simulink model "LRSim1D_V3"  (R2016b)
settings: Solver=ode45  StartTime=0  StopTime=tend  FixedStep=0.005  RelTol=1e-4
values from neighbouring files (symbols this model uses):
  g = 9.81    [EnginePerformance.m]    (also in LaunchControl.m; runsim.m)
undefined symbols (not defined in the file or in its folder): Eng, Prop, Roc
settings Model: Creator=adamb  LastModifiedBy=adamb
settings SolverCC: ZeroCrossAlgorithm=Adaptive

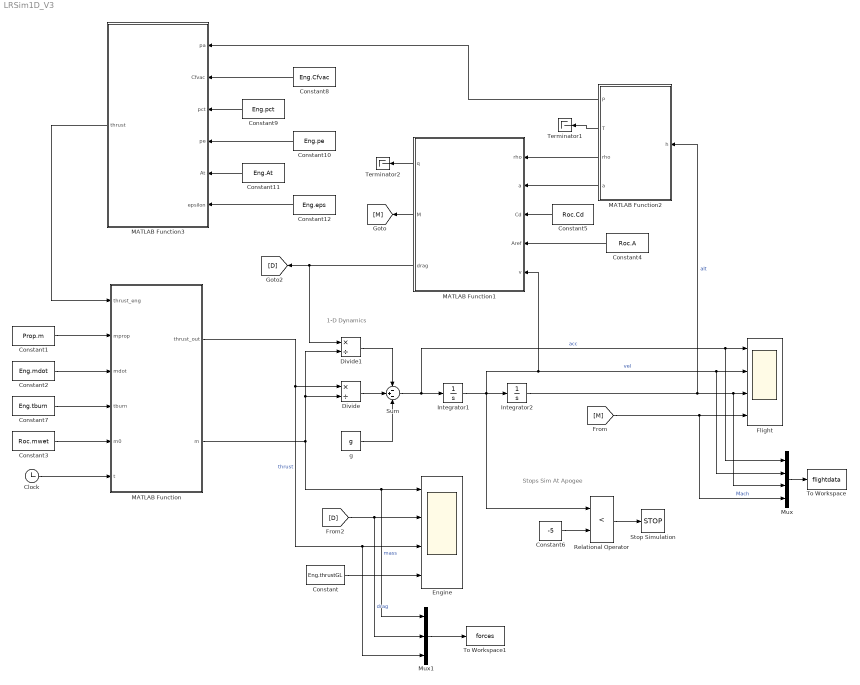
== system LRSim1D_V3 ==
  note: Stops Sim At Apogee
  note: 1-D Dynamics
  Clock : Clock
  Constant : Constant  Value=Eng.thrustGL
  Constant1 : Constant  Value=Prop.m
  Constant10 : Constant  Value=Eng.pe
  Constant11 : Constant  Value=Eng.At
  Constant12 : Constant  Value=Eng.eps
  Constant2 : Constant  Value=Eng.mdot
  Constant3 : Constant  Value=Roc.mwet
  Constant4 : Constant  Value=Roc.A
  Constant5 : Constant  Value=Roc.Cd  VectorParams1D=off
  Constant6 : Constant  Value=-5
  Constant7 : Constant  Value=Eng.tburn
  Constant8 : Constant  Value=Eng.Cfvac
  Constant9 : Constant  Value=Eng.pct
  Divide : Product  Inputs=*/
  Divide1 : Product  Inputs=*/
  Engine : Scope  NumInputPorts=4
  Flight : Scope  NumInputPorts=4
  Integrator1 : Integrator
  Integrator2 : Integrator
  MATLAB Function : MATLAB Function  TreatAsAtomicUnit=on
  MATLAB Function1 : MATLAB Function  TreatAsAtomicUnit=on
  MATLAB Function2 : MATLAB Function  TreatAsAtomicUnit=on
  MATLAB Function3 : MATLAB Function  TreatAsAtomicUnit=on
  Mux : Mux
  Mux1 : Mux  Inputs=3
  Relational Operator : RelationalOperator  Operator=<  OutDataTypeStr=boolean  RndMeth=Simplest
  Stop Simulation : Stop
  Sum : Sum  Inputs=-+-
  Terminator1 : Terminator
  Terminator2 : Terminator
  To Workspace : ToWorkspace  VariableName=flightdata  SampleTime=-1
  To Workspace1 : ToWorkspace  VariableName=forces  SampleTime=-1
  g : Constant  Value=g
  wires:
  Sum/1 -> Mux/1, Flight/1, Integrator1/1  "acc"
  MATLAB Function3/1(thrust) -> MATLAB Function/1(thrust_eng)
  Constant1/1 -> MATLAB Function/2(mprop)
  Constant3/1 -> MATLAB Function/5(m0)
  Constant2/1 -> MATLAB Function/3(mdot)
  Clock/1 -> MATLAB Function/6(t)
  MATLAB Function/2(m) -> Divide1/2, Divide/2, Mux1/1, Engine/1  "mass"
  MATLAB Function/1(thrust_out) -> Mux1/3, Engine/3, Divide/1  "thrust"
  Integrator1/1 -> Relational Operator/1, Mux/2, Flight/2, MATLAB Function1/5(v), Integrator2/1  "vel"
  Integrator2/1 -> MATLAB Function2/1(h), Mux/3, Flight/3  "alt"
  Divide/1 -> Sum/2
  g/1 -> Sum/3
  Constant4/1 -> MATLAB Function1/4(Aref)
  Constant5/1 -> MATLAB Function1/3(Cd)
  MATLAB Function1/2(M) -> [M]
  [M] -> Mux/4, Flight/4  "Mach"
  MATLAB Function1/3(drag) -> [D], Divide1/1
  Divide1/1 -> Sum/1
  Relational Operator/1 -> Stop Simulation/1
  Constant6/1 -> Relational Operator/2
  MATLAB Function2/4(a) -> MATLAB Function1/2(a)
  MATLAB Function2/3(rho) -> MATLAB Function1/1(rho)
  Constant7/1 -> MATLAB Function/4(tburn)
  MATLAB Function2/1(P) -> MATLAB Function3/1(pa)
  Constant9/1 -> MATLAB Function3/3(pct)
  Constant10/1 -> MATLAB Function3/4(pe)
  Constant11/1 -> MATLAB Function3/5(At)
  Constant12/1 -> MATLAB Function3/6(epsilon)
  Mux/1 -> To Workspace/1
  Constant8/1 -> MATLAB Function3/2(Cfvac)
  MATLAB Function2/2(T) -> Terminator1/1
  Constant/1 -> Engine/4
  [D] -> Mux1/2, Engine/2  "drag"
  Mux1/1 -> To Workspace1/1
  MATLAB Function1/1(q) -> Terminator2/1

== matlab function LRSim1D_V3/MATLAB Function1 ==
  data: rho input; a input; q output; M output; Cd input; Aref input; v input; drag output
function [q,M,drag] = AeroComputation(rho,a,Cd,Aref,v)

M = abs(v/a); % Mach #
q = 0.5*rho*abs(v)*v; % qbar, Dynamic Pressure

A = Aref(1);
CdM = interp1(Cd(1,:),Cd(2,:),M); % Interpolates the Cd based on M

drag = q*A*CdM;


end

== matlab function LRSim1D_V3/MATLAB Function ==
  data: thrust_eng input; thrust_out output; mprop input; mdot input; tburn input; m0 input; t input; m output
function [thrust_out,m] = FlightComputer(thrust_eng,mprop,mdot,tburn,...
                      m0,t)

% This determines mass, thrust, and staging
% Don't worry about this part
% Thrust has a smooth rise and fall for discrete integration
if t<0
    thrust_out = 0;
    m = m0;
elseif t > tburn
    thrust_out = 0;
    m = m0-mprop;
else
    m = m0 - mdot*t;
    % Thrust function
    if t <= 0.2
        t = t-0.1;
        thrust_out = thrust_eng*(1/(1+exp(-100*t)));
    elseif t > 0.2 && t <= (tburn-0.2)
        thrust_out = thrust_eng;
    else
        t = t - (tburn-0.2) - 0.1;
        thrust_out = thrust_eng*(1/(1+exp(100*t)));
    end    
end

end

== matlab function LRSim1D_V3/MATLAB Function2 ==
  data: h input; P output; T output; rho output; a output
function [P,T,rho,a] = AtmosParams(h)

[P,rho,T,a] = StdAtmos(h);

end

== matlab function LRSim1D_V3/MATLAB Function3 ==
  data: pa input; Cfvac input; pct input; pe input; At input; thrust output; epsilon input
function thrust  = ThrustCalc(pa,Cfvac,pct,pe,At,epsilon)

% Actual thrust coefficient 
Cf = Cfvac + (epsilon*At)*((pe-pa)/pct);
% Output thrust
thrust = pct*At*Cf; % [N]

end
